simulink library "slident"  (Simulink 5.0)
values from neighbouring files (symbols this model uses):
  A = s(1:2,1:2)    [motor.m]
  B = s(1:2,3)    [motor.m]
  C = eye(2)    [motor.m]
  D = D .* abs(ec{kexp}*ones(1,size(D,2)))    [arx.m]    (also in motor.m = [0;0])
  data = iddata(data,[],T)    [ar.m]    (also in arx.m = complex(data); idfilt.m = zfc{1}; pem.m = pvset(data,'Name',inputname(1)); predict.m = nkshift(data,Inpd,'append'))
  ts = ts{1}    [arx.m]    (also in idfilt.m = pvget(data,'Ts'))
  Ts = pvget(m0,'Ts')    [arx.m]    (also in idfilt.m = {1}; n4sid_f.m = {Ts}; predict.m = [])
  X0 = [0;0]    [motor.m]    (also in predict.m = X0*ones(1,Ne))
  z = ze{kexp}    [arx.m]    (also in arxstruc.m; bj.m = pvset(z,'Name',inputname(1)); idfilt.m = zc{kexp}; ivstruc.m)
undefined symbols (not defined in the file or in its folder): Demos, idss, offset, ph, slident2, Tdi, tsn
libraries: simulink x1
settings Model: RequirementInfo=9  Creator=greg  LastModifiedBy=jglass

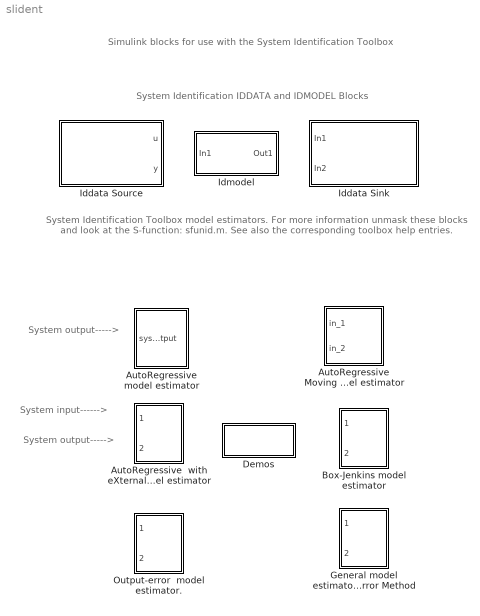
== system slident ==
  note: System Identification IDDATA and IDMODEL Blocks
  note: System output----->
  note: System input------>
  note: System output----->
  note: System Identification Toolbox
      | model estimators. For more information
      | unmask these blocks and look at the
      | S-function: sfunid.m.
      | See also the corresponding toolbox
      | help entries.
  note: Simulink blocks for use with
      | the System Identification Toolbox
  AutoRegressive model estimator : Subsystem  AncestorBlock=slident2/AutoRegressive model estimator  mask(AR){order=3, HowOften=25, tso=0.05, npts=200, mn=, cbsim=1 step prediction}
      mask prompts: order "Orders of model [na]:"; HowOften "How often update model (samples)"; tso "Sample time:"; npts "Length of Data Window"; mn "Model Name"; cbsim "Prediction horizon"
      mask help:
      | Autoregressive model estimator for a scalar valued signal
      | Hook input 1 to the signal
      | Model Name: Enter workspace variable name for resulting models.Leave empty for printout on screen.
      | Choose predictionhorizon for the plots.
      mask init:
      | method='ar';
      | [ts,offset,ph,mn]=slidentinit(tso,cbsim,mn);
      mask Help:
      | Hook the signal to the input of this block.
      | The estimated models are based on the latest data in the Data window. (initially padded
      | with zeros).
      | The model is reestimated at the chosen rate. <p>
      | 
      | If a Model Name M is entered, the variable M will contain the estimated models
      | in a cell array, so that M{k,1} is the time associated with the the k:th model and
      | M{k,2} is the actual model in IDPOLY format. The models can be investigated by
      | all the usual commands in the ident toolbox. For example, bode(M{:;2}) and
      | step(M{:,2}) will show the bode plots and step responses of all the models.
      | <p>
      | If the model name is left empty, the models will be written to the command screen.
      | <p>
      | The properties of the models will also be displayed, on-line, as the  predicted
      | output of the current model,compared with the measured, actual output. Choose
      |  between various prediction horizons.
      | 
      | Results are displayed as the one step ahead predicted output versus the true output in graphical form.
      mask StyleString: edit,edit,edit,edit,edit,popup(1 step prediction|5 step prediction|10 step prediction)
      mask Display:
      | disp('AR')
      | port_label('input',1,'y')
  AutoRegressive  with eXternal input model estimator : Subsystem  AncestorBlock=|  mask(ARX){order=[2 2 1], HowOften=25, tso=0.05, npts=200, mn=, cbsim=Simulation}
      | slident2/AutoRegressive 
      | with eXternal input
      | model estimator
      mask prompts: order "Orders of model [na nb nk]:"; HowOften "How often update model (samples)"; tso "Sample time:"; npts "Length of Data window"; mn "Model Name"; cbsim "Simulation/Prediction"
      mask help:
      | ARX model estimator.
      | Hook input 1 to system input.
      | Hook input 2 to system output.
      | Model Name: Enter workspace variable name for resulting models. Leave empty for printout on screen.
      | Choose if presented model plots should be simulation or prediction.
      mask init:
      | method='arx';
      | [ts,offset,ph,mn]=slidentinit(tso,cbsim,mn);
      mask Help:
      | Hook the system's input to the first port of this block and the system's
      |  output to second port.
      | The estimated models are based on the latest data in the Data window. (initially padded
      | with zeros).
      | The model is reestimated at the chosen rate. <p>
      | 
      | If a Model Name M is entered, the variable M will contain the estimated models
      | in a cell array, so that M{k,1} is the time associated with the the k:th model and
      | M{k,2} is the actual model in IDPOLY format. The models can be investigated by
      | all the usual commands in the ident toolbox. For example, bode(M{:;2}) and
      | step(M{:,2}) will show the bode plots and step responses of all the models.
      | <p>
      | If the model name is left empty, the models will be written to the command screen.
      | <p>
      | The properties of the models will also be displayed, on-line, as the simulated/predicted
      | output of the current model,compared with the measured, actual output. Choose between
      | simulated outputs and predicted outputs over various prediction horizons.
      mask StyleString: edit,edit,edit,edit,edit,popup(Simulation|1 step prediction|5 step prediction|10 step prediction)
      mask Display:
      | disp('ARX')
      | port_label('input',1,'u')
      | port_label('input',2,'y')
  AutoRegressive Moving Average with eXternal input model estimator : Subsystem  AncestorBlock=|  mask(ARMAX){order=[2 2 2 1], HowOften=25, tso=0.05, npts=200, mn=, cbsim=Simulation}
      | slident2/AutoRegressive Moving
      | Average with eXternal
      | input model estimator
      mask prompts: order "Orders of model [na nb nc nk]"; HowOften "Calculate after how many points:"; tso "Sample time:"; npts "Length of Data Window"; mn "Model Name"; cbsim "Simulation/Prediction"
      mask help:
      | ARMAX model estimator.
      | Hook input 1 to system input.
      | Hook input 2 to system output.
      | Model Name: Enter workspace variable name for resulting models.Leave empty for printout on screen.
      | Choose if presented model plots should be simulation or prediction.
      mask init:
      | method='armax';
      | [ts,offset,ph,mn]=slidentinit(tso,cbsim,mn);
      mask Help:
      | Hook the system's input to the first port of this block and the system's
      |  output to second port.
      | The estimated models are based on the latest data in the Data window. (initially padded
      | with zeros).
      | The model is reestimated at the chosen rate. <p>
      | 
      | If a Model Name M is entered, the variable M will contain the estimated models
      | in a cell array, so that M{k,1} is the time associated with the the k:th model and
      | M{k,2} is the actual model in IDPOLY format. The models can be investigated by
      | all the usual commands in the ident toolbox. For example, bode(M{:;2}) and
      | step(M{:,2}) will show the bode plots and step responses of all the models.
      | <p>
      | If the model name is left empty, the models will be written to the command screen.
      | <p>
      | The properties of the models will also be displayed, on-line, as the simulated/predicted
      | output of the current model,compared with the measured, actual output. Choose between
      | simulated outputs and predicted outputs over various prediction horizons.
      mask StyleString: edit,edit,edit,edit,edit,popup(Simulation|1 step prediction|5 step prediction|10 step prediction)
      mask Display:
      | disp('ARMAX')
      | port_label('input',1,'u')
      | port_label('input',2,'y')
  Box-Jenkins model estimator : Subsystem  AncestorBlock=slident2/Box-Jenkins model estimator  mask(BJ){order=[2 2 2 2 1], HowOften=25, tso=0.05, npts=200, mn=, cbsim=Simulation}
      mask prompts: order "Orders of model [na nc nd nf nk]"; HowOften "Calculate after how many points:"; tso "Sample time:"; npts "Length of Data Window"; mn "Model Name"; cbsim "Simulation/Prediction"
      mask help:
      | Box-Jenkins model estimator.
      | Hook input 1 to system input.
      | Hook input 2 to system output.
      | Model Name: Enter workspace variable name for resulting models.Leave empty for printout on screen.
      | Choose if presented model plots should be simulation or prediction.
      mask init:
      | method='bj';
      | [ts,offset,ph,mn]=slidentinit(tso,cbsim,mn);
      mask Help:
      | Hook the system's input to the first port of this block and the system's
      |  output to second port.
      | The estimated models are based on the latest data in the Data window. (initially padded
      | with zeros).
      | The model is reestimated at the chosen rate. <p>
      | 
      | If a Model Name M is entered, the variable M will contain the estimated models
      | in a cell array, so that M{k,1} is the time associated with the the k:th model and
      | M{k,2} is the actual model in IDPOLY format. The models can be investigated by
      | all the usual commands in the ident toolbox. For example, bode(M{:;2}) and
      | step(M{:,2}) will show the bode plots and step responses of all the models.
      | <p>
      | If the model name is left empty, the models will be written to the command screen.
      | <p>
      | The properties of the models will also be displayed, on-line, as the simulated/predicted
      | output of the current model,compared with the measured, actual output. Choose between
      | simulated outputs and predicted outputs over various prediction horizons.
      mask StyleString: edit,edit,edit,edit,edit,popup(Simulation|1 step prediction|5 step prediction|10 step prediction)
      mask Display:
      | disp('BJ')
      | port_label('input',1,'u')
      | port_label('input',2,'y')
  Demos : Subsystem  AncestorBlock=slident2/Demos
      settings: OpenFcn=demo toolbox
      mask Display: disp('Demos')
  General model estimator using Predictive Error Method : Subsystem  AncestorBlock=|  mask(PEM){order=[2 2 2 2 2 1], HowOften=25, tso=0.05, npts=200, mn=, cbsim=Simulation}
      | slident2/General model
      | estimator using
      | Predictive Error Method
      mask prompts: order "Orders of model [na nb nc nd nf nk]:"; HowOften "Calculate after how many points:"; tso "Sample time:"; npts "Length of Data Window"; mn "Model Name"; cbsim "Simulation/Prediction"
      mask help:
      | General SISO polynomial model estimator.
      | Hook input 1 to system input.
      | Hook input 2 to system output.
      | Model Name: Enter workspace variable name for resulting models.Leave empty for printout on screen.
      | Choose if presented model plots should be simulation or prediction. .
      mask init:
      | method='pem';
      | [ts,offset,ph,mn]=slidentinit(tso,cbsim,mn);
      mask Help:
      | Hook the system's input to the first port of this block and the system's
      |  output to second port.
      | The estimated models are based on the latest data in the Data window. (initially padded
      | with zeros).
      | The model is reestimated at the chosen rate. <p>
      | 
      | If a Model Name M is entered, the variable M will contain the estimated models
      | in a cell array, so that M{k,1} is the time associated with the the k:th model and
      | M{k,2} is the actual model in IDPOLY format. The models can be investigated by
      | all the usual commands in the ident toolbox. For example, bode(M{:;2}) and
      | step(M{:,2}) will show the bode plots and step responses of all the models.
      | <p>
      | If the model name is left empty, the models will be written to the command screen.
      | <p>
      | The properties of the models will also be displayed, on-line, as the simulated/predicted
      | output of the current model,compared with the measured, actual output. Choose between
      | simulated outputs and predicted outputs over various prediction horizons.
      mask StyleString: edit,edit,edit,edit,edit,popup(Simulation|1 step prediction|5 step prediction|10 step prediction)
      mask Display:
      | disp('PEM')
      | port_label('input',1,'u')
      | port_label('input',2,'y')
  Iddata Sink : Subsystem  mask(IDDATA Sink){name=data, Ts=0.1}
      mask prompts: name "IDDATA Name"; Ts "Sample Time (sec.)"
      mask help: Enter in a name of a variable for which you would like the IDDATA data object be saved. The sample time is the rate that the data will be sampled.
      mask Help:
      | Enter in a name of a variable for which you would like the IDDATA data object be saved.
      | 
      | The sample time is the rate that the data will be sampled.
      mask Display:
      | disp('IDDATA SINK')
      | port_label('input',1,'Input')
      | port_label('input',2,'Output')
  Iddata Source : Subsystem  AncestorBlock=slident/Iddata Input Output  mask(Iddata InputOutput){iddataobj=z}
      mask prompts: iddataobj "Iddata object"
      mask help:
      | This block allows to import IDDATA object from the main work space of Matlab.
      |
      | The first output port of the block corresponds to the input signal of the IDDATA object and the second output port corresponds to the output signal.
      |
      | Enter an IDDATA object in the dialog field.
      mask init:
      | Ts=iddataobj.Ts;
      | TimeUnit=iddataobj.TimeUnit;  if isempty(TimeUnit), TimeUnit='s'; end
      | if lower(TimeUnit(1))=='m', Ts=Ts*60;
      | elseif  lower(TimeUnit(1))=='h', Ts=Ts*3600;
      | end
      mask Help:
      | This block allows to import IDDATA object from the main work space of Matlab.
      | <p>
      | The output port of the block corresponds to the input signal of the IDDATA object.
      | <p>
      | Enter an IDDATA object in the dialog field.
      | <p>
      | Use the block IDDATA Input for the input data only.
      mask Display:
      | disp('IDDATA SOURCE')
      | port_label('output',1,'Input')
      | port_label('output',2,'Output')
  "Idmodel " : Subsystem  mask(Idmodel Block){sys=idss(-1,1,1,0), IC=0, noi=on, seed=}
      mask prompts: sys "idmodel variable"; IC "Initial state (state space only: 'z', 'm', or vector )"; noi "Add noise"; seed "Noise seed(s).  Default empty"
      mask help:
      | Enter any Idmodel object (Idpoly, Idss, Idarx, Idgrey or Idproc).
      | For simulations  with noise, Seed(s) may be left empty for random restarts.
      | Enter as many seeds as there are outputs for specific realizations.
      mask init:
      | [A,B,C,D,Ts,Tdi,X0,tsn,variance,ActSeed,sysname]=idmdlmask('InitializeData',gcb,sys,IC,noi,seed);
      | idmdlmask('UpdateDiagram',gcb,Ts,noi);
      mask Help:
      | The IDMODEL  block 	accepts any IDMODEL defined in the System Identification Toolbox: IDPOLY, IDSS,
      | IDGREY, IDARX and IDPROC. <p><P>
      | 
      | In the editiable text box enter the name of any IDMODEL in workspace.<p><p>
      | 
      |  For IDMODELS in state-space (IDSS and IDGREY) the initial state vector may be
      | specified. Use 'z' (within quotes) or 0 for zero initial conditions, use 'm' for the
      | Model's own initial state (I.e. MOD.X0) or specify the initial state  as a vector.<p><p>
      | 
      | To add noise to the simulation, check the corresponding box. Noise will be
      | added in accordance with the models noise specifications, i.e. MOD.NoiseVariance and
      | the matrices or polynomials that determine the color of the additive noise. <p><p>
      | 
      | For continuous time models the variance of the momentary noise term is infinite
      | in theory. You will see an appropriately bandlimited version, taking into account
      | the natural time constants of the system. You may think of the resulting simulated output
      | being filtered with a low-pass filter with a pass-band that does not distort the dynamics
      | from the input.<p><p>
      | 
      | IDMODELS with time-delays (MOD.InputDelay nonzero) are properly treated. Discrete time
      | models are convereted into models which take care of the delay explicitly, (thereby
      | extending also X0). For continuous time models a transport delay block is used.
      mask CallbackString: idmdlmask('MaskLTICallback',gcb)||idmdlmask('MaskLTICallback',gcb)|
      mask Display: disp(sysname)
  Output-error  model estimator. : Subsystem  AncestorBlock="slident2/Output-error  model estimator."  mask(OE){order=[2 2 1], HowOften=25, tso=0.05, npts=200, mn=, cbsim=Simulation}
      mask prompts: order "Orders of model [nb nf nk]:"; HowOften "How often update model"; tso "Sample time:"; npts "Length of Data Window"; mn "Model Name"; cbsim "Simulation/Prediction"
      mask help:
      | Output-error model estimator.
      | Hook input 1 to system input.
      | Hook input 2 to system output.
      | Model Name: Enter workspace variable name for resulting models.Leave empty for printout on screen.
      | Choose if presented model plots should be simulation or prediction.
      mask init:
      | method='oe';
      | [ts,offset,ph,mn]=slidentinit(tso,cbsim,mn);
      mask Help:
      | Hook the system's input to the first port of this block and the system's
      |  output to second port.
      | The estimated models are based on the latest data in the Data window. (initially padded
      | with zeros).
      | The model is reestimated at the chosen rate. <p>
      | 
      | If a Model Name M is entered, the variable M will contain the estimated models
      | in a cell array, so that M{k,1} is the time associated with the the k:th model and
      | M{k,2} is the actual model in IDPOLY format. The models can be investigated by
      | all the usual commands in the ident toolbox. For example, bode(M{:;2}) and
      | step(M{:,2}) will show the bode plots and step responses of all the models.
      | <p>
      | If the model name is left empty, the models will be written to the command screen.
      | <p>
      | The properties of the models will also be displayed, on-line, as the simulated/predicted
      | output of the current model,compared with the measured, actual output. Choose between
      | simulated outputs and predicted outputs over various prediction horizons.
      mask StyleString: edit,edit,edit,edit,edit,popup(Simulation|1 step prediction|5 step prediction|10 step prediction)
      mask Display:
      | disp('OE')
      | port_label('input',1,'u')
      | port_label('input',2,'y')

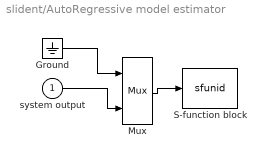
== system slident/AutoRegressive model estimator ==
  system output : Inport
  Ground : Ground
  Mux : Mux  Inputs=2
  S-function block : S-Function  FunctionName=sfunid  Parameters=order,npts,HowOften,offset,ts,method,mn,ph
      settings: DeleteFcn=sfunid([],[],[],'DeleteBlock')
  wires:
  Ground/1 -> Mux/1
  system output/1 -> Mux/2
  Mux/1 -> S-function block/1

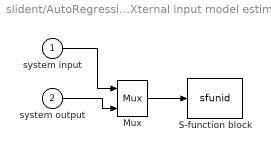
== system slident/AutoRegressive  with eXternal input model estimator ==
  system input : Inport
  system output : Inport  Port=2
  Mux : Mux  Inputs=2
  S-function block : S-Function  FunctionName=sfunid  Parameters=order,npts,HowOften,offset,ts,method,mn,ph
      settings: DeleteFcn=sfunid([],[],[],'DeleteBlock')
  wires:
  system input/1 -> Mux/1
  system output/1 -> Mux/2
  Mux/1 -> S-function block/1

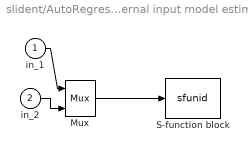
== system slident/AutoRegressive Moving Average with eXternal input model estimator ==
  in_1 : Inport
  in_2 : Inport  Port=2
  Mux : Mux  Inputs=2
  S-function block : S-Function  FunctionName=sfunid  Parameters=order,npts,HowOften,offset,ts,method,mn,ph
      settings: DeleteFcn=sfunid([],[],[],'DeleteBlock')
  wires:
  Mux/1 -> S-function block/1
  in_1/1 -> Mux/1
  in_2/1 -> Mux/2

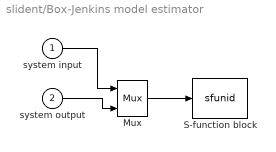
== system slident/Box-Jenkins model estimator ==
  system input : Inport
  system output : Inport  Port=2
  Mux : Mux  Inputs=2
  S-function block : S-Function  FunctionName=sfunid  Parameters=order,npts,HowOften,offset,ts,method,mn,ph
      settings: DeleteFcn=sfunid([],[],[],'DeleteBlock')
  wires:
  Mux/1 -> S-function block/1
  system output/1 -> Mux/2
  system input/1 -> Mux/1

== system slident/Demos ==

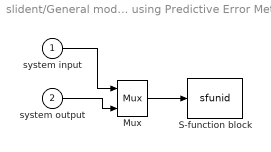
== system slident/General model estimator using Predictive Error Method ==
  system input : Inport
  system output : Inport  Port=2
  Mux : Mux  Inputs=2
  S-function block : S-Function  FunctionName=sfunid  Parameters=order,npts,HowOften,offset,ts,method,mn,ph
      settings: DeleteFcn=sfunid([],[],[],'DeleteBlock')
  wires:
  Mux/1 -> S-function block/1
  system output/1 -> Mux/2
  system input/1 -> Mux/1

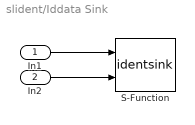
== system slident/Iddata Sink ==
  In1 : Inport
  In2 : Inport  Port=2
  S-Function : S-Function  FunctionName=identsink  Parameters=name Ts
  wires:
  In2/1 -> S-Function/2
  In1/1 -> S-Function/1

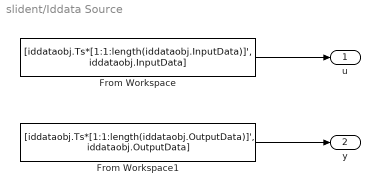
== system slident/Iddata Source ==
  From Workspace : FromWorkspace  VariableName=[iddataobj.Ts*[1:1:length(iddataobj.InputData)]', iddataobj.InputData]  SampleTime=Ts  Interpolate=off  OutputAfterFinalValue=Setting to zero
  From Workspace1 : FromWorkspace  VariableName=[iddataobj.Ts*[1:1:length(iddataobj.OutputData)]', iddataobj.OutputData]  SampleTime=Ts  Interpolate=off  OutputAfterFinalValue=Setting to zero
  u : Outport
  y : Outport  Port=2
  wires:
  From Workspace/1 -> u/1
  From Workspace1/1 -> y/1

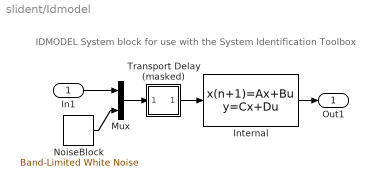
== system slident/Idmodel  ==
  note: IDMODEL System block
      | for use with the
      | System Identification Toolbox
  In1 : Inport
  Internal : DiscreteStateSpace  A=A  B=B  C=C  D=D  X0=X0  SampleTime=Ts
  Mux : Mux  Inputs=2
  NoiseBlock : simulink/Sources/Band-Limited White Noise  Tag=NoiseBlock  Cov=variance  Ts=tsn  seed=ActSeed
  Transport Delay (masked) : Subsystem  Tag=InputDelayBlock  AncestorBlock=|  mask(Transport Delay (masked)){Td=Tdi, u0=0, bufsize=1024}
      | identextras/Transport Delay
      | (masked)
      mask prompts: Td "Delay Time"; u0 "Initial Input"; bufsize "Initial Buffer Size"
      mask help: Transport Delay, with direct feedthrough when Delay Time is equal to zero.
      mask init:
      | df = get_param(bdroot,'dirty');
      | iddfthru(gcb, Td, u0, bufsize);
      | set_param(bdroot,'dirty',df)
      mask Help: See Transport Delay for more information.
      mask Display: block_icon('Transport Delay')
  Out1 : Outport
  wires:
  Transport Delay (masked)/1(Outport) -> Internal/1
  Mux/1 -> Transport Delay (masked)/1(Inport)
  Internal/1 -> Out1/1
  In1/1 -> Mux/1
  NoiseBlock/1 -> Mux/2

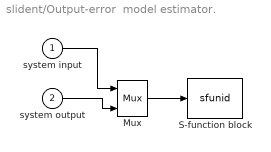
== system slident/Output-error  model estimator. ==
  system input : Inport
  system output : Inport  Port=2
  Mux : Mux  Inputs=2
  S-function block : S-Function  FunctionName=sfunid  Parameters=order,npts,HowOften,offset,ts,method,mn,ph
      settings: DeleteFcn=sfunid([],[],[],'DeleteBlock')
  wires:
  system input/1 -> Mux/1
  system output/1 -> Mux/2
  Mux/1 -> S-function block/1

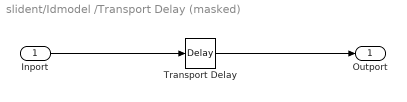
== system slident/Idmodel /Transport Delay (masked) ==
  Inport : Inport
  Transport Delay : TransportDelay  DelayTime=0.147909753458958
  Outport : Outport
  wires:
  Transport Delay/1 -> Outport/1
  Inport/1 -> Transport Delay/1
